simulink model "Control_test"  (R2014b)
settings: Solver=FixedStepDiscrete  StartTime=0.0  StopTime=Inf  FixedStep=0.001  RelTol=1e-3
PostLoadFcn:
  | , if any(exist('dsrtsu_mdlpostloadfcn', 'file') == [2, 3, 6]), try dsrtsu_mdlpostloadfcn('Execute', bdroot); catch fprintf('Error in PostLoadFcn (dsrtsu_mdlpostloadfcn) for model "%s":\n %s\n', bdroot, lasterr); end, end,
undefined symbols (not defined in the file or in its folder): dtLocal, slcm
libraries: rtican x163, simulink x14
(part 31 of 34)

== system Control_test/InputProcessing/VehicleCanProcessing/EMS2 ==
  Bus Creator : BusCreator  Inputs=19
  L_EMS2 : rtican/RTICAN Receive (RX)   Reserved1=[]  Reserved2=[]  Reserved3=[]  Reserved4=[]  SfcnMessage=[]  Msg_Struct=[]  BoardTypeNo=[]  BoardNo=[]  ChannelNo=[]  Parameters=[]  DialogFcn=[]  UnitName=[]  Revision=[]  UnitValues=[]  DSProperties=struct('RTI',struct('Version',uint32(5),'BlockType',struct('isSLSource',uint8(1),'isSLSink',uint8(1),'isHWSource',uint8(0),'isHWSink',uint8(0),'isSetup',uint8(0),'isInline',uint8(1),'isNonInline',uint8(0),'isInterrupt',uint8(0),'isChannelwise',uint8(0)),'IOBoardType','RTICAN','UnitType','MESSAGE','Identifier','RX','DialogType','MSVC','BlockSet','RTICAN','SlaveProcessor','CAN'))  RTIBlockInterface=struct('OutputPortsWidth',int32([1 1 1 1 1 1 1 1 1 1 1 1 1 1 1 1 1 1 1]),'OutputPortsActive',[1 1 1 1 1 1 1 1 1 1 1 1 1 1 1 1 1 1 1],'OutputPortsName',{{'PV_AV_CAN','TEMP_ENG','MAF_FAC_ALTI_MMV','VB_OFF_ACT','GP_CTL','CLU_ACK','OD_OFF_REQ','BRAKE_ACT','ACK_ES','ENG_CHR','CONF_MIL_FMY','ACC_ACT','TPS','ENG_VOL','MUL_CODE','CAN_VERS','CONF_TCU','OBD_FRF_ACK','TQ_STND'}},'OutputPortsDataType',{{'SS_DOUBLE','SS_DOUBLE','SS_DOUBLE','SS_DOUBLE','SS_DOUBLE','SS_DOUBLE','SS_DOUBLE','SS_DOUBLE','SS_DOUBLE','SS_DOUBLE','SS_DOUBLE','SS_DOUBLE','SS_DOUBLE','SS_DOUBLE','SS_DOUBLE','SS_DOUBLE','SS_DOUBLE','SS_DOUBLE','SS_DOUBLE'}},'OutputPortsLabel',{{'PV_AV_CAN','TEMP_ENG','MAF_FAC_ALTI_MMV','VB_OFF_ACT','GP_CTL','CLU_ACK','OD_OFF_REQ','BRAKE_ACT','ACK_ES','ENG_CHR','CONF_MIL_FMY','ACC_ACT','TPS','ENG_VOL','MUL_CODE','CAN_VERS','CONF_TCU','OBD_FRF_ACK','TQ_STND'}},'OutputPortsLabelMode','ON','InputPortsWidth',int32(0),'InputPortsActive',0,'DialogFcn','rtican_message_interface_gui','BlockDisplay',{{'','center'}},'IconTransparency','on','ParameterTunableNames',{{}},'InitLevel',3,'BlockName',struct('Token',{{'L_EMS2'}}),'SampleTime',{{-1}},'TriggerPort',{{'none'}},'EnablePort',{{'none'}})  RTIBlockParameters=struct('BoardTypeNo',{{1,'OFF',[]}},'BoardNo',{{1,'ON',[1 16]}},'ChannelNo',{{1,'ON',[1 2]}},'Parameters',{{struct('DataFileSupport',struct('DataFileSelectedMaster',1,'DataFileSelectedLocal',1,'DataFileName','c:\users\mpc_car\documents\github\mpc-car\controller\dbcfiles\hmc_can_for_ucb_v1.dbc|','DataFileDate',['21-Nov-2014 13:30:51'],'SelectedFile','c:\users\mpc_car\documents\github\mpc-car\dbcfiles\hmc_can_for_ucb_v2.dbc','InterfaceFcn','rtican_dbc_file_parser'),'Options',struct('StatusSelected',0,'TimeSelected',0,'DeltaTimeSelected',0,'BytePortSelected',0,'MessageLengthSelected',0,'TriggerPort',struct('Selected',0,'TriggerType',0),'UserCoding',struct('Selected',0,'InterfaceFile','UserDecodingFile','FcnName','UserDecodeFcn','InportSelected',0,'InportWidth',1,'OutportSelected',0,'OutportWidth',1),'EnablePortSelected',0,'SignalOnPortnameSelected',1,'UseRXService',0),'Message',struct('MsgOnBlocknameSelected',1,'MsgName','L_EMS2','MsgIdFormat',0,'MsgId',515,'MsgLength',8,'NumSignals',19,'SampleTime',-1,'Signal',struct('SgnName',{'PV_AV_CAN','TEMP_ENG','MAF_FAC_ALTI_MMV','VB_OFF_ACT','GP_CTL','CLU_ACK','OD_OFF_REQ','BRAKE_ACT','ACK_ES','ENG_CHR','CONF_MIL_FMY','ACC_ACT','TPS','ENG_VOL','MUL_CODE','CAN_VERS','CONF_TCU','OBD_FRF_ACK','TQ_STND'},'SgnStartBit',{0,8,16,24,25,27,28,29,31,32,36,39,40,48,56,58,58,58,58},'SgnLength',{8,8,8,1,2,1,1,2,1,4,3,1,8,8,2,6,6,6,6},'ByteLayout',{0,0,0,0,0,0,0,0,0,0,0,0,0,0,0,0,0,0,0},'Factor',{0.3906,0.75,0.00781,1,1,1,1,1,1,1,1,1,0.4694836,0.1,1,1,1,1,10},'Offset',{0,-48,0,0,0,0,0,0,0,0,0,0,-15.0234742,0,0,0,0,0,0},'SgnComment',{['In case of Delphi ECU, Output period tolerance(+1ms) will be applied to Engine Lamda3.'],['In case of Delphi ECU, Output period tolerance(+1ms) will be applied to Engine Lamda3.'],['In case of Delphi ECU, Output period tolerance(+1ms) will be applied to Engine Lamda3.'],['1. This signal is only for the gasoline system.' char(10) '2. In case of Delphi ECU, Output period tolerance(+1ms) will be applied to Engine Lamda3.'],['1. This signal is for the diesel engine system only.' char(10) '2. In case of Delphi ECU, Output period tolerance(+1ms) will be applied to Engine Lamda3.'],['1. This signal is for the diesel engine and ISG system installed vehicles only.' char(10) '2. In case of Delphi ECU, Output period tolerance(+1ms) will be applied to Engine Lamda3.'],['1. This signal is available in the auto cruise control system equiped vehicles only.' char(10) '2. In case of Delphi ECU, Output period tolerance(+1ms) will be applied to Engine Lamda3.'],['In case of Delphi ECU, Output period tolerance(+1ms) will be applied to Engine Lamda3.'],['In case of Delphi ECU, Output period tolerance(+1ms) will be applied to Engine Lamda3.'],['1. For the automatic variant coding at E.O.L : This signal value is valid 1.5sec later from initial IG-ON' char(10) '2. In case of Delphi ECU, Output period tolerance(+1ms) will be applied to Engine Lamda3.'],['1. This value represents a calibrated constant from the ECU.' char(10) '2. In case of Delphi ECU, Output period tolerance(+1ms) will be applied to Engine Lamda3.'],['1. There is signal relationship between ¡®ACC_ACT¡¯ and ¡®PV_AV_CAN¡¯. See ¡®PV_AV_CAN¡¯ signal description page.' char(10) '2. In case of Delphi ECU, Output period tolerance(+1ms) will be applied to Engine Lamda3.'],['1. In diesel engine system, there is a signal relationship between TPS and PV_AV_CAN. For the details, please see PV_AV_CAN signal description page. ' char(10) '2. In case of Delphi ECU, Output period tolerance(+1ms) will be applied to Engine Lamda3.'],['In case of Delphi ECU, Output period tolerance(+1ms) will be applied to Engine Lamda3.'],['In case of Delphi ECU, Output period tolerance(+1ms) will be applied to Engine Lamda3.'],['In case of Delphi ECU, Output period tolerance(+1ms) will be applied to Engine Lamda3.'],['1. For the automatic variant coding at E.O.L : This signal value is valid 1.5sec later from initial IG-ON' char(10) '2. In case of Delphi ECU, Output period tolerance(+1ms) will be applied to Engine Lamda3.'],['In case of Delphi ECU, Output period tolerance(+1ms) will be applied to Engine Lamda3.'],['1. In case of an engine which maximum engine torque is higher than 520Nm, this factor value is 15.' char(10) '2. In case of Delphi ECU, Output period tolerance(+1ms) will be applied to Engine Lamda3.']},'SgnUnit',{'%','¡É','','','','','','','','','','','%','liter','','','','','Nm'},'Min',{0,-48,0,0,0,0,0,0,0,0,0,0,-15.0234742,0,0,0,0,0,0},'Max',{99.603,143.25,1.99155,1,3,1,1,3,1,15,7,1,104.6948357,25.5,3,7.7,63,63,630},'SgnType',{0,0,0,0,0,0,0,0,0,0,0,0,0,0,1,2,2,2,2},'SLDataType',{'SS_DOUBLE','SS_DOUBLE','SS_DOUBLE','SS_DOUBLE','SS_DOUBLE','SS_DOUBLE','SS_DOUBLE','SS_DOUBLE','SS_DOUBLE','SS_DOUBLE','SS_DOUBLE','SS_DOUBLE','SS_DOUBLE','SS_DOUBLE','SS_DOUBLE','SS_DOUBLE','SS_DOUBLE','SS_DOUBLE','SS_DOUBLE'},'DataType',{0,0,0,0,0,0,0,0,0,0,0,0,0,0,0,0,0,0,0},'ModeValue',{-1,-1,-1,-1,-1,-1,-1,-1,-1,-1,-1,-1,-1,-1,-1,0,1,2,3}),'MsgIdNumFormat',0,'MsgComment',{{''}}),'Version',1.2,'general',struct('isFromLib',0)),'OFF',[]}},'GroupId',{{struct('Group',{{'RTICAN'}},'No',1,'Behavior',{{'NAMECHANGE'}},'BlockType',{{'SINK'}},'NameChangeFlag',0),'OFF',[]}},'SFcnRTICANMessage',{{struct('MsgType','RX','SFcnPortType','Scalar','MsgName','L_EMS2','MsgIdFormat','STD','MsgId',515,'MsgLength',8,'NumSignals',19,'SampleTime',-1,'Signal',struct('SgnName',{'PV_AV_CAN','TEMP_ENG','MAF_FAC_ALTI_MMV','VB_OFF_ACT','GP_CTL','CLU_ACK','OD_OFF_REQ','BRAKE_ACT','ACK_ES','ENG_CHR','CONF_MIL_FMY','ACC_ACT','TPS','ENG_VOL','MUL_CODE','CAN_VERS','CONF_TCU','OBD_FRF_ACK','TQ_STND'},'SgnStartBit',{0,8,16,24,25,27,28,29,31,32,36,39,40,48,56,58,58,58,58},'SgnLength',{8,8,8,1,2,1,1,2,1,4,3,1,8,8,2,6,6,6,6},'ByteLayout',{['little endian'],['little endian'],['little endian'],['little endian'],['little endian'],['little endian'],['little endian'],['little endian'],['little endian'],['little endian'],['little endian'],['little endian'],['little endian'],['little endian'],['little endian'],['little endian'],['little endian'],['little endian'],['little endian']},'Factor',{0.3906,0.75,0.00781,1,1,1,1,1,1,1,1,1,0.4694836,0.1,1,1,1,1,10},'Offset',{0,-48,0,0,0,0,0,0,0,0,0,0,-15.0234742,0,0,0,0,0,0},'SgnType',{'standard','standard','standard','standard','standard','standard','standard','standard','standard','standard','standard','standard','standard','standard','mode','mode-dependent','mode-dependent','mode-dependent','mode-dependent'},'SLDataType',{'SS_DOUBLE','SS_DOUBLE','SS_DOUBLE','SS_DOUBLE','SS_DOUBLE','SS_DOUBLE','SS_DOUBLE','SS_DOUBLE','SS_DOUBLE','SS_DOUBLE','SS_DOUBLE','SS_DOUBLE','SS_DOUBLE','SS_DOUBLE','SS_DOUBLE','SS_DOUBLE','SS_DOUBLE','SS_DOUBLE','SS_DOUBLE'},'DataType',{['unsigned int'],['unsigned int'],['unsigned int'],['unsigned int'],['unsigned int'],['unsigned int'],['unsigned int'],['unsigned int'],['unsigned int'],['unsigned int'],['unsigned int'],['unsigned int'],['unsigned int'],['unsigned int'],['unsigned int'],['unsigned int'],['unsigned int'],['unsigned int'],['unsigned int']},'ModeValue',{-1,-1,-1,-1,-1,-1,-1,-1,-1,-1,-1,-1,-1,-1,-1,0,1,2,3}),'StatusSelected','no','TimeSelected','no','DeltaTimeSelected','no','BytePortSelected','no','MessageLengthSelected','no','TriggerPort',struct('Selected','no','TriggerType',0),'UserCoding',struct('Selected','no','InterfaceFile','UserDecodingFile','FcnName','UserDecodeFcn','InportSelected','no','InportWidth',1,'OutportSelected','no','OutportWidth',1),'EnablePortSelected','no','UseRXService','no','BoardType','DS1','BoardNo',1,'ControllerNo',1),'OFF',[]}},'TLCFileName',{{'rtican_rx_message','OFF',[]}})  RTISFcnParameters=struct('SFcnRTICANMessage','struct','TLCFileName','char')  RTIBlockParaDefault=struct('BoardTypeNo',4302,'BoardNo',1,'ChannelNo',1,'Parameters',struct('DataFileSupport',struct('DataFileSelectedMaster',0,'DataFileSelectedLocal',0,'DataFileName','','DataFileDate','','SelectedFile',['<no file selected>']),'Options',struct('StatusSelected',1,'TimeSelected',1,'DeltaTimeSelected',1,'BytePortSelected',0,'MessageLengthSelected',0,'TriggerPort',struct('Selected',0,'TriggerType','rising'),'UserCoding',struct('Selected',0,'InterfaceFile','UserDecodingFile','FcnName','UserDecodeFcn','InportSelected',0,'InportWidth',1,'OutportSelected',0,'OutportWidth',1),'EnablePortSelected',0,'SignalOnPortnameSelected',1,'UseRXService',0),'Message',struct('MsgOnBlocknameSelected',0,'MsgName',['RX Message'],'MsgIdFormat',0,'MsgId',100,'MsgLength',8,'NumSignals',1,'SampleTime',-1,'Signal',struct('SgnName',['RX signal'],'SgnStartBit',0,'SgnLength',8,'SgnType',0,'ModeValue',-1,'DataType',0,'SLDataType','SS_DOUBLE','ByteLayout',0,'Factor',1,'Offset',0,'Min',0,'Max',255,'SgnComment',{{}},'SgnUnit',''),'MsgIdNumFormat',0,'MsgComment',{{''}}),'Version',1.2,'general',struct('isFromLib',1)),'GroupId',struct('Group',{{'RTICAN'}},'No',1,'Behavior',{{'NAMECHANGE'}},'BlockType',{{'SINK'}},'NameChangeFlag',0),'SFcnRTICANMessage',struct('MsgType','RX','MsgName',['RX Message'],'MsgIdFormat','STD','MsgId',100,'MsgLength',8,'NumSignals',1,'SampleTime',-1,'Signal',struct('SgnName',['RX signal'],'SgnStartBit',0,'SgnLength',8,'SgnType','standard','ModeValue',-1,'DataType',['unsigned int'],'ByteLayout',['little endian'],'SLDataType','SS_DOUBLE','Factor',1,'Offset',0),'StatusSelected','yes','TimeSelected','yes','DeltaTimeSelected','yes','BytePortSelected','no','MessageLengthSelected','no','EnablePortSelected','no','UserCoding',struct('Selected','no','InterfaceFile','UserDecodingFile','FcnName','UserDecodeFcn','InportSelected','no','InportWidth',1,'OutportSelected','no','OutportWidth',1),'TriggerPort',struct('Selected','no','TriggerType','rising'),'UseRXService','no','BoardType','DS4302','BoardNo',1,'ControllerNo',1,'SFcnPortType','Scalar'),'TLCFileName','rtican_rx_message')
      settings: AttributesFormatString=Group Id: RTICAN1\n
  EMS2_CAN : Outport
  wires:
  Bus Creator/1 -> EMS2_CAN/1  "EMS2_CAN"
  L_EMS2/1 -> Bus Creator/1  "PV_AV_CAN"
  L_EMS2/2 -> Bus Creator/2  "TEMP_ENG"
  L_EMS2/3 -> Bus Creator/3  "MAF_FAC_ALTI_MMV"
  L_EMS2/4 -> Bus Creator/4  "VB_OFF_ACT"
  L_EMS2/5 -> Bus Creator/5  "GP_CTL"
  L_EMS2/6 -> Bus Creator/6  "CLU_ACK"
  L_EMS2/7 -> Bus Creator/7  "OD_OFF_REQ"
  L_EMS2/8 -> Bus Creator/8  "BRAKE_ACT"
  L_EMS2/9 -> Bus Creator/9  "ACK_ES"
  L_EMS2/10 -> Bus Creator/10  "ENG_CHR"
  L_EMS2/11 -> Bus Creator/11  "CONF_MIL_FMY"
  L_EMS2/12 -> Bus Creator/12  "ACC_ACT"
  L_EMS2/13 -> Bus Creator/13  "TPS"
  L_EMS2/14 -> Bus Creator/14  "ENG_VOL"
  L_EMS2/15 -> Bus Creator/15  "MUL_CODE"
  L_EMS2/16 -> Bus Creator/16  "CAN_VERS"
  L_EMS2/17 -> Bus Creator/17  "CONF_TCU"
  L_EMS2/18 -> Bus Creator/18  "OBD_FRF_ACK"
  L_EMS2/19 -> Bus Creator/19  "TQ_STND"

== system Control_test/InputProcessing/VehicleCanProcessing/ESP2 ==
  Bus Creator : BusCreator  Inputs=12
  L_ESP2 : rtican/RTICAN Receive (RX)   Reserved1=[]  Reserved2=[]  Reserved3=[]  Reserved4=[]  SfcnMessage=[]  Msg_Struct=[]  BoardTypeNo=[]  BoardNo=[]  ChannelNo=[]  Parameters=[]  DialogFcn=[]  UnitName=[]  Revision=[]  UnitValues=[]  DSProperties=struct('RTI',struct('Version',uint32(5),'BlockType',struct('isSLSource',uint8(1),'isSLSink',uint8(1),'isHWSource',uint8(0),'isHWSink',uint8(0),'isSetup',uint8(0),'isInline',uint8(1),'isNonInline',uint8(0),'isInterrupt',uint8(0),'isChannelwise',uint8(0)),'IOBoardType','RTICAN','UnitType','MESSAGE','Identifier','RX','DialogType','MSVC','BlockSet','RTICAN','SlaveProcessor','CAN'))  RTIBlockInterface=struct('OutputPortsWidth',int32([1 1 1 1 1 1 1 1 1 1 1 1]),'OutputPortsActive',[1 1 1 1 1 1 1 1 1 1 1 1],'OutputPortsName',{{'LAT_ACCEL','LONG_ACCEL_STAT','LAT_ACCEL_STAT','LONG_ACCEL_DIAG','CYL_PRES_STAT','CYL_PRESS_DIAG','YAW_RATE','YAW_RATE_STAT','LAT_ACCEL_DIAG','YAW_RATE_DIAG','LONG_ACCEL','CYL_PRES'}},'OutputPortsDataType',{{'SS_DOUBLE','SS_DOUBLE','SS_DOUBLE','SS_DOUBLE','SS_DOUBLE','SS_DOUBLE','SS_DOUBLE','SS_DOUBLE','SS_DOUBLE','SS_DOUBLE','SS_DOUBLE','SS_DOUBLE'}},'OutputPortsLabel',{{'LAT_ACCEL','LONG_ACCEL_STAT','LAT_ACCEL_STAT','LONG_ACCEL_DIAG','CYL_PRES_STAT','CYL_PRESS_DIAG','YAW_RATE','YAW_RATE_STAT','LAT_ACCEL_DIAG','YAW_RATE_DIAG','LONG_ACCEL','CYL_PRES'}},'OutputPortsLabelMode','ON','InputPortsWidth',int32(0),'InputPortsActive',0,'DialogFcn','rtican_message_interface_gui','BlockDisplay',{{'','center'}},'IconTransparency','on','ParameterTunableNames',{{}},'InitLevel',3,'BlockName',struct('Token',{{'L_ESP2'}}),'SampleTime',{{-1}},'TriggerPort',{{'none'}},'EnablePort',{{'none'}})  RTIBlockParameters=struct('BoardTypeNo',{{1,'OFF',[]}},'BoardNo',{{1,'ON',[1 16]}},'ChannelNo',{{1,'ON',[1 2]}},'Parameters',{{struct('DataFileSupport',struct('DataFileSelectedMaster',1,'DataFileSelectedLocal',1,'DataFileName','c:\users\mpc_car\documents\github\mpc-car\controller\dbcfiles\hmc_can_for_ucb_v1.dbc|','DataFileDate',['21-Nov-2014 13:30:51'],'SelectedFile','c:\users\mpc_car\documents\github\mpc-car\dbcfiles\hmc_can_for_ucb_v2.dbc','InterfaceFcn','rtican_dbc_file_parser'),'Options',struct('StatusSelected',0,'TimeSelected',0,'DeltaTimeSelected',0,'BytePortSelected',0,'MessageLengthSelected',0,'TriggerPort',struct('Selected',0,'TriggerType',0),'UserCoding',struct('Selected',0,'InterfaceFile','UserDecodingFile','FcnName','UserDecodeFcn','InportSelected',0,'InportWidth',1,'OutportSelected',0,'OutportWidth',1),'EnablePortSelected',0,'SignalOnPortnameSelected',1,'UseRXService',0),'Message',struct('MsgOnBlocknameSelected',1,'MsgName','L_ESP2','MsgIdFormat',0,'MsgId',516,'MsgLength',8,'NumSignals',12,'SampleTime',-1,'Signal',struct('SgnName',{'LAT_ACCEL','LONG_ACCEL_STAT','LAT_ACCEL_STAT','LONG_ACCEL_DIAG','CYL_PRES_STAT','CYL_PRESS_DIAG','YAW_RATE','YAW_RATE_STAT','LAT_ACCEL_DIAG','YAW_RATE_DIAG','LONG_ACCEL','CYL_PRES'},'SgnStartBit',{0,11,12,13,14,15,16,29,30,31,32,48},'SgnLength',{11,1,1,1,1,1,13,1,1,1,11,12},'ByteLayout',{0,0,0,0,0,0,0,0,0,0,0,0},'Factor',{0.01,1,1,1,1,1,0.01,1,1,1,0.01,0.1},'Offset',{-10.23,0,0,0,0,0,-40.95,0,0,0,-10.23,0},'SgnComment',{'','','','','','','','','','','',''},'SgnUnit',{'m/s^2','','','','','','¢ª/s','','','','m/s^2','bar'},'Min',{-10.23,0,0,0,0,0,-40.95,0,0,0,-10.23,0},'Max',{10.24,1,1,1,1,1,40.96,1,1,1,10.24,409.5},'SgnType',{0,0,0,0,0,0,0,0,0,0,0,0},'SLDataType',{'SS_DOUBLE','SS_DOUBLE','SS_DOUBLE','SS_DOUBLE','SS_DOUBLE','SS_DOUBLE','SS_DOUBLE','SS_DOUBLE','SS_DOUBLE','SS_DOUBLE','SS_DOUBLE','SS_DOUBLE'},'DataType',{0,0,0,0,0,0,0,0,0,0,0,0},'ModeValue',{-1,-1,-1,-1,-1,-1,-1,-1,-1,-1,-1,-1}),'MsgIdNumFormat',0,'MsgComment',{{''}}),'Version',1.2,'general',struct('isFromLib',0)),'OFF',[]}},'GroupId',{{struct('Group',{{'RTICAN'}},'No',1,'Behavior',{{'NAMECHANGE'}},'BlockType',{{'SINK'}},'NameChangeFlag',0),'OFF',[]}},'SFcnRTICANMessage',{{struct('MsgType','RX','SFcnPortType','Scalar','MsgName','L_ESP2','MsgIdFormat','STD','MsgId',516,'MsgLength',8,'NumSignals',12,'SampleTime',-1,'Signal',struct('SgnName',{'LAT_ACCEL','LONG_ACCEL_STAT','LAT_ACCEL_STAT','LONG_ACCEL_DIAG','CYL_PRES_STAT','CYL_PRESS_DIAG','YAW_RATE','YAW_RATE_STAT','LAT_ACCEL_DIAG','YAW_RATE_DIAG','LONG_ACCEL','CYL_PRES'},'SgnStartBit',{0,11,12,13,14,15,16,29,30,31,32,48},'SgnLength',{11,1,1,1,1,1,13,1,1,1,11,12},'ByteLayout',{['little endian'],['little endian'],['little endian'],['little endian'],['little endian'],['little endian'],['little endian'],['little endian'],['little endian'],['little endian'],['little endian'],['little endian']},'Factor',{0.01,1,1,1,1,1,0.01,1,1,1,0.01,0.1},'Offset',{-10.23,0,0,0,0,0,-40.95,0,0,0,-10.23,0},'SgnType',{'standard','standard','standard','standard','standard','standard','standard','standard','standard','standard','standard','standard'},'SLDataType',{'SS_DOUBLE','SS_DOUBLE','SS_DOUBLE','SS_DOUBLE','SS_DOUBLE','SS_DOUBLE','SS_DOUBLE','SS_DOUBLE','SS_DOUBLE','SS_DOUBLE','SS_DOUBLE','SS_DOUBLE'},'DataType',{['unsigned int'],['unsigned int'],['unsigned int'],['unsigned int'],['unsigned int'],['unsigned int'],['unsigned int'],['unsigned int'],['unsigned int'],['unsigned int'],['unsigned int'],['unsigned int']},'ModeValue',{-1,-1,-1,-1,-1,-1,-1,-1,-1,-1,-1,-1}),'StatusSelected','no','TimeSelected','no','DeltaTimeSelected','no','BytePortSelected','no','MessageLengthSelected','no','TriggerPort',struct('Selected','no','TriggerType',0),'UserCoding',struct('Selected','no','InterfaceFile','UserDecodingFile','FcnName','UserDecodeFcn','InportSelected','no','InportWidth',1,'OutportSelected','no','OutportWidth',1),'EnablePortSelected','no','UseRXService','no','BoardType','DS1','BoardNo',1,'ControllerNo',1),'OFF',[]}},'TLCFileName',{{'rtican_rx_message','OFF',[]}})  RTISFcnParameters=struct('SFcnRTICANMessage','struct','TLCFileName','char')  RTIBlockParaDefault=struct('BoardTypeNo',4302,'BoardNo',1,'ChannelNo',1,'Parameters',struct('DataFileSupport',struct('DataFileSelectedMaster',0,'DataFileSelectedLocal',0,'DataFileName','','DataFileDate','','SelectedFile',['<no file selected>']),'Options',struct('StatusSelected',1,'TimeSelected',1,'DeltaTimeSelected',1,'BytePortSelected',0,'MessageLengthSelected',0,'TriggerPort',struct('Selected',0,'TriggerType','rising'),'UserCoding',struct('Selected',0,'InterfaceFile','UserDecodingFile','FcnName','UserDecodeFcn','InportSelected',0,'InportWidth',1,'OutportSelected',0,'OutportWidth',1),'EnablePortSelected',0,'SignalOnPortnameSelected',1,'UseRXService',0),'Message',struct('MsgOnBlocknameSelected',0,'MsgName',['RX Message'],'MsgIdFormat',0,'MsgId',100,'MsgLength',8,'NumSignals',1,'SampleTime',-1,'Signal',struct('SgnName',['RX signal'],'SgnStartBit',0,'SgnLength',8,'SgnType',0,'ModeValue',-1,'DataType',0,'SLDataType','SS_DOUBLE','ByteLayout',0,'Factor',1,'Offset',0,'Min',0,'Max',255,'SgnComment',{{}},'SgnUnit',''),'MsgIdNumFormat',0,'MsgComment',{{''}}),'Version',1.2,'general',struct('isFromLib',1)),'GroupId',struct('Group',{{'RTICAN'}},'No',1,'Behavior',{{'NAMECHANGE'}},'BlockType',{{'SINK'}},'NameChangeFlag',0),'SFcnRTICANMessage',struct('MsgType','RX','MsgName',['RX Message'],'MsgIdFormat','STD','MsgId',100,'MsgLength',8,'NumSignals',1,'SampleTime',-1,'Signal',struct('SgnName',['RX signal'],'SgnStartBit',0,'SgnLength',8,'SgnType','standard','ModeValue',-1,'DataType',['unsigned int'],'ByteLayout',['little endian'],'SLDataType','SS_DOUBLE','Factor',1,'Offset',0),'StatusSelected','yes','TimeSelected','yes','DeltaTimeSelected','yes','BytePortSelected','no','MessageLengthSelected','no','EnablePortSelected','no','UserCoding',struct('Selected','no','InterfaceFile','UserDecodingFile','FcnName','UserDecodeFcn','InportSelected','no','InportWidth',1,'OutportSelected','no','OutportWidth',1),'TriggerPort',struct('Selected','no','TriggerType','rising'),'UseRXService','no','BoardType','DS4302','BoardNo',1,'ControllerNo',1,'SFcnPortType','Scalar'),'TLCFileName','rtican_rx_message')
      settings: AttributesFormatString=Group Id: RTICAN1\n
  ESP2_CAN : Outport
  wires:
  Bus Creator/1 -> ESP2_CAN/1  "ESP2_CAN"
  L_ESP2/1 -> Bus Creator/1  "LAT_ACCEL"
  L_ESP2/2 -> Bus Creator/2  "LONG_ACCEL_STAT"
  L_ESP2/3 -> Bus Creator/3  "LAT_ACCEL_STAT"
  L_ESP2/4 -> Bus Creator/4  "LONG_ACCEL_DIAG"
  L_ESP2/5 -> Bus Creator/5  "CYL_PRES_STAT"
  L_ESP2/6 -> Bus Creator/6  "CYL_PRESS_DIAG"
  L_ESP2/7 -> Bus Creator/7  "YAW_RATE"
  L_ESP2/8 -> Bus Creator/8  "YAW_RATE_STAT"
  L_ESP2/9 -> Bus Creator/9  "LAT_ACCEL_DIAG"
  L_ESP2/10 -> Bus Creator/10  "YAW_RATE_DIAG"
  L_ESP2/11 -> Bus Creator/11  "LONG_ACCEL"
  L_ESP2/12 -> Bus Creator/12  "CYL_PRES"

== system Control_test/InputProcessing/VehicleCanProcessing/ESP2Processing ==
  In1 : Inport
  Bus Creator3 : BusCreator  Inputs=12
  Bus Selector3 : BusSelector  OutputSignals=LAT_ACCEL,LAT_ACCEL_STAT,LAT_ACCEL_DIAG,LONG_ACCEL,LONG_ACCEL_STAT,LONG_ACCEL_DIAG,CYL_PRES,CYL_PRES_STAT,CYL_PRESS_DIAG,YAW_RATE,YAW_RATE_STAT,YAW_RATE_DIAG
  ESP2 Processing : Subsystem
  Out1 : Outport
  tag scope: ipLongAccel=global
  wires:
  Bus Selector3/1 -> ESP2 Processing/1(LAT_ACCEL_CAN)  "<LAT_ACCEL>"
  Bus Selector3/2 -> ESP2 Processing/2(LAT_ACCEL_STAT_CAN)  "<LAT_ACCEL_STAT>"
  Bus Selector3/3 -> ESP2 Processing/3(LAT_ACCEL_DIAG_CAN)  "<LAT_ACCEL_DIAG>"
  Bus Selector3/4 -> ESP2 Processing/4(LONG_ACCEL_CAN)  "<LONG_ACCEL>"
  Bus Selector3/5 -> ESP2 Processing/5(LONG_ACCEL_STAT_CAN)  "<LONG_ACCEL_STAT>"
  Bus Selector3/6 -> ESP2 Processing/6(LONG_ACCEL_DIAG_CAN)  "<LONG_ACCEL_DIAG>"
  Bus Selector3/7 -> ESP2 Processing/7(CYL_PRES_CAN)  "<CYL_PRES>"
  Bus Selector3/8 -> ESP2 Processing/8(CYL_PRES_STAT_CAN)  "<CYL_PRES_STAT>"
  Bus Selector3/9 -> ESP2 Processing/9(CYL_PRES_DIAG_CAN)  "<CYL_PRESS_DIAG>"
  Bus Selector3/10 -> ESP2 Processing/10(YAW_RATE_CAN)  "<YAW_RATE>"
  Bus Selector3/11 -> ESP2 Processing/11(YAW_RATE_STAT_CAN)  "<YAW_RATE_STAT>"
  Bus Selector3/12 -> ESP2 Processing/12(YAW_RATE_DIAG_CAN)  "<YAW_RATE_DIAG>"
  ESP2 Processing/1(ipLatAccel [m/s2]) -> Bus Creator3/1
  ESP2 Processing/2(ipLatAccelFail) -> Bus Creator3/2
  ESP2 Processing/3(ipLatAccelDiag) -> Bus Creator3/3
  ESP2 Processing/4(ipLongAccel [m/s2]) -> [ipLongAccel], Bus Creator3/4
  ESP2 Processing/5(ipLongAccelFail) -> Bus Creator3/5
  ESP2 Processing/6(ipLongAccelDiag) -> Bus Creator3/6
  ESP2 Processing/7(ipMsCylPress [bar]) -> Bus Creator3/7
  ESP2 Processing/8(ipMsCylPressFail) -> Bus Creator3/8
  ESP2 Processing/9(ipMsCylPressDiag) -> Bus Creator3/9
  ESP2 Processing/10(ipYawRate [deg/s]) -> Bus Creator3/10
  ESP2 Processing/11(ipYawRateFail) -> Bus Creator3/11
  ESP2 Processing/12(ipYawRateDiag) -> Bus Creator3/12
  Bus Creator3/1 -> Out1/1  "ESP2Data"
  In1/1 -> Bus Selector3/1

== system Control_test/InputProcessing/VehicleCanProcessing/MDPS2 ==
  Bus Creator : BusCreator  Inputs=5
  L_MDPS2 : rtican/RTICAN Receive (RX)   Reserved1=[]  Reserved2=[]  Reserved3=[]  Reserved4=[]  SfcnMessage=[]  Msg_Struct=[]  BoardTypeNo=[]  BoardNo=[]  ChannelNo=[]  Parameters=[]  DialogFcn=[]  UnitName=[]  Revision=[]  UnitValues=[]  DSProperties=struct('RTI',struct('Version',uint32(5),'BlockType',struct('isSLSource',uint8(1),'isSLSink',uint8(1),'isHWSource',uint8(0),'isHWSink',uint8(0),'isSetup',uint8(0),'isInline',uint8(1),'isNonInline',uint8(0),'isInterrupt',uint8(0),'isChannelwise',uint8(0)),'IOBoardType','RTICAN','UnitType','MESSAGE','Identifier','RX','DialogType','MSVC','BlockSet','RTICAN','SlaveProcessor','CAN'))  RTIBlockInterface=struct('OutputPortsWidth',int32([1 1 1 1 1]),'OutputPortsActive',[1 1 1 1 1],'OutputPortsName',{{'CR_Mdps_DrvTq','CR_Mdps_StrAng','CF_Mdps_AliveCnt','CF_Mdps_Stat','CF_Mdps_Chksum'}},'OutputPortsDataType',{{'SS_DOUBLE','SS_DOUBLE','SS_DOUBLE','SS_DOUBLE','SS_DOUBLE'}},'OutputPortsLabel',{{'CR_Mdps_DrvTq','CR_Mdps_StrAng','CF_Mdps_AliveCnt','CF_Mdps_Stat','CF_Mdps_Chksum'}},'OutputPortsLabelMode','ON','InputPortsWidth',int32(0),'InputPortsActive',0,'DialogFcn','rtican_message_interface_gui','BlockDisplay',{{'','center'}},'IconTransparency','on','ParameterTunableNames',{{}},'InitLevel',3,'BlockName',struct('Token',{{'L_MDPS2'}}),'SampleTime',{{-1}},'TriggerPort',{{'none'}},'EnablePort',{{'none'}})  RTIBlockParameters=struct('BoardTypeNo',{{1,'OFF',[]}},'BoardNo',{{1,'ON',[1 16]}},'ChannelNo',{{1,'ON',[1 2]}},'Parameters',{{struct('DataFileSupport',struct('DataFileSelectedMaster',1,'DataFileSelectedLocal',1,'DataFileName',['c:\users\mpc lab\documents\github\controller\dbcfiles\hmc_can_for_ucb_v2.dbc|'],'DataFileDate',{{{['10-Feb-2015 13:24:58']}}},'SelectedFile','..\..\..\dbcfiles\hmc_can_for_ucb_v2.dbc','InterfaceFcn','rtican_dbc_file_parser'),'Options',struct('StatusSelected',0,'TimeSelected',0,'DeltaTimeSelected',0,'BytePortSelected',0,'MessageLengthSelected',0,'TriggerPort',struct('Selected',0,'TriggerType',0),'UserCoding',struct('Selected',0,'InterfaceFile','UserDecodingFile','FcnName','UserDecodeFcn','InportSelected',0,'InportWidth',1,'OutportSelected',0,'OutportWidth',1),'EnablePortSelected',0,'SignalOnPortnameSelected',1,'UseRXService',0),'Message',struct('MsgOnBlocknameSelected',1,'MsgName','L_MDPS2','MsgIdFormat',0,'MsgId',517,'MsgLength',8,'NumSignals',5,'SampleTime',-1,'Signal',struct('SgnName',{'CR_Mdps_DrvTq','CR_Mdps_StrAng','CF_Mdps_AliveCnt','CF_Mdps_Stat','CF_Mdps_Chksum'},'SgnStartBit',{0,16,40,48,56},'SgnLength',{12,16,8,4,8},'SgnType',{0,0,0,0,0},'ModeValue',{-1,-1,-1,-1,-1},'DataType',{0,1,0,0,0},'ByteLayout',{0,0,0,0,0},'Factor',{0.01,0.1,1,1,1},'Offset',{-20.48,0,0,0,0},'SgnComment',{{''},{''},{''},{''},{''}},'SgnUnit',{'','Degree','','',''},'Min',{-20.48,-3276.8,0,0,0},'Max',{20.46,3276.7,255,15,255},'SLDataType',{'SS_DOUBLE','SS_DOUBLE','SS_DOUBLE','SS_DOUBLE','SS_DOUBLE'}),'MsgIdNumFormat',0,'MsgComment',{{''}}),'Version',1.2,'general',struct('isFromLib',0)),'OFF',[]}},'GroupId',{{struct('Group',{{'RTICAN'}},'No',1,'Behavior',{{'NAMECHANGE'}},'BlockType',{{'SINK'}},'NameChangeFlag',0),'OFF',[]}},'SFcnRTICANMessage',{{struct('MsgType','RX','SFcnPortType','Scalar','MsgName','L_MDPS2','MsgIdFormat','STD','MsgId',517,'MsgLength',8,'NumSignals',5,'SampleTime',-1,'Signal',struct('SgnName',{'CR_Mdps_DrvTq','CR_Mdps_StrAng','CF_Mdps_AliveCnt','CF_Mdps_Stat','CF_Mdps_Chksum'},'SgnStartBit',{0,16,40,48,56},'SgnLength',{12,16,8,4,8},'SgnType',{'standard','standard','standard','standard','standard'},'ModeValue',{-1,-1,-1,-1,-1},'DataType',{['unsigned int'],['signed int'],['unsigned int'],['unsigned int'],['unsigned int']},'ByteLayout',{['little endian'],['little endian'],['little endian'],['little endian'],['little endian']},'Factor',{0.01,0.1,1,1,1},'Offset',{-20.48,0,0,0,0},'SLDataType',{'SS_DOUBLE','SS_DOUBLE','SS_DOUBLE','SS_DOUBLE','SS_DOUBLE'}),'StatusSelected','no','TimeSelected','no','DeltaTimeSelected','no','BytePortSelected','no','MessageLengthSelected','no','TriggerPort',struct('Selected','no','TriggerType',0),'UserCoding',struct('Selected','no','InterfaceFile','UserDecodingFile','FcnName','UserDecodeFcn','InportSelected','no','InportWidth',1,'OutportSelected','no','OutportWidth',1),'EnablePortSelected','no','UseRXService','no','BoardType','DS1','BoardNo',1,'ControllerNo',1),'OFF',[]}},'TLCFileName',{{'rtican_rx_message','OFF',[]}})  RTISFcnParameters=struct('SFcnRTICANMessage','struct','TLCFileName','char')  RTIBlockParaDefault=struct('BoardTypeNo',4302,'BoardNo',1,'ChannelNo',1,'Parameters',struct('DataFileSupport',struct('DataFileSelectedMaster',0,'DataFileSelectedLocal',0,'DataFileName','','DataFileDate','','SelectedFile',['<no file selected>']),'Options',struct('StatusSelected',1,'TimeSelected',1,'DeltaTimeSelected',1,'BytePortSelected',0,'MessageLengthSelected',0,'TriggerPort',struct('Selected',0,'TriggerType','rising'),'UserCoding',struct('Selected',0,'InterfaceFile','UserDecodingFile','FcnName','UserDecodeFcn','InportSelected',0,'InportWidth',1,'OutportSelected',0,'OutportWidth',1),'EnablePortSelected',0,'SignalOnPortnameSelected',1,'UseRXService',0),'Message',struct('MsgOnBlocknameSelected',0,'MsgName',['RX Message'],'MsgIdFormat',0,'MsgId',100,'MsgLength',8,'NumSignals',1,'SampleTime',-1,'Signal',struct('SgnName',['RX signal'],'SgnStartBit',0,'SgnLength',8,'SgnType',0,'ModeValue',-1,'DataType',0,'SLDataType','SS_DOUBLE','ByteLayout',0,'Factor',1,'Offset',0,'Min',0,'Max',255,'SgnComment',{{}},'SgnUnit',''),'MsgIdNumFormat',0,'MsgComment',{{''}}),'Version',1.2,'general',struct('isFromLib',1)),'GroupId',struct('Group',{{'RTICAN'}},'No',1,'Behavior',{{'NAMECHANGE'}},'BlockType',{{'SINK'}},'NameChangeFlag',0),'SFcnRTICANMessage',struct('MsgType','RX','MsgName',['RX Message'],'MsgIdFormat','STD','MsgId',100,'MsgLength',8,'NumSignals',1,'SampleTime',-1,'Signal',struct('SgnName',['RX signal'],'SgnStartBit',0,'SgnLength',8,'SgnType','standard','ModeValue',-1,'DataType',['unsigned int'],'ByteLayout',['little endian'],'SLDataType','SS_DOUBLE','Factor',1,'Offset',0),'StatusSelected','yes','TimeSelected','yes','DeltaTimeSelected','yes','BytePortSelected','no','MessageLengthSelected','no','EnablePortSelected','no','UserCoding',struct('Selected','no','InterfaceFile','UserDecodingFile','FcnName','UserDecodeFcn','InportSelected','no','InportWidth',1,'OutportSelected','no','OutportWidth',1),'TriggerPort',struct('Selected','no','TriggerType','rising'),'UseRXService','no','BoardType','DS4302','BoardNo',1,'ControllerNo',1,'SFcnPortType','Scalar'),'TLCFileName','rtican_rx_message')
      settings: AttributesFormatString=Group Id: RTICAN1\n
  MDPS2_CAN : Outport
  wires:
  Bus Creator/1 -> MDPS2_CAN/1  "MDPS2"
  L_MDPS2/1 -> Bus Creator/1  "CR_Mdps_DrvTq"
  L_MDPS2/2 -> Bus Creator/2  "CR_Mdps_StrAng"
  L_MDPS2/3 -> Bus Creator/3  "CF_Mdps_AliveCnt"
  L_MDPS2/4 -> Bus Creator/4  "CF_Mdps_Stat"
  L_MDPS2/5 -> Bus Creator/5  "CF_Mdps_Chksum"

== system Control_test/InputProcessing/VehicleCanProcessing/MDPS2 Processing ==
  In1 : Inport
  Out1 : Outport
  wires:
  In1/1 -> Out1/1  "MDPS2Data"

== system Control_test/InputProcessing/VehicleCanProcessing/MDPS3 ==
  Bus Creator : BusCreator  Inputs=7
  L_MDPS3 : rtican/RTICAN Receive (RX)   Reserved1=[]  Reserved2=[]  Reserved3=[]  Reserved4=[]  SfcnMessage=[]  Msg_Struct=[]  BoardTypeNo=[]  BoardNo=[]  ChannelNo=[]  Parameters=[]  DialogFcn=[]  UnitName=[]  Revision=[]  UnitValues=[]  DSProperties=struct('RTI',struct('Version',uint32(5),'BlockType',struct('isSLSource',uint8(1),'isSLSink',uint8(1),'isHWSource',uint8(0),'isHWSink',uint8(0),'isSetup',uint8(0),'isInline',uint8(1),'isNonInline',uint8(0),'isInterrupt',uint8(0),'isChannelwise',uint8(0)),'IOBoardType','RTICAN','UnitType','MESSAGE','Identifier','RX','DialogType','MSVC','BlockSet','RTICAN','SlaveProcessor','CAN'))  RTIBlockInterface=struct('OutputPortsWidth',int32([1 1 1 1 1 1 1]),'OutputPortsActive',[1 1 1 1 1 1 1],'OutputPortsName',{{'CF_Mdps_MsgCount3','CR_Mdps_StrColTq','CF_Mdps_ToiFlt','CF_Mdps_ToiActive','CF_Mdps_FailStat','CF_Mdps_ToiUnavail','CF_Mdps_Chksum3'}},'OutputPortsDataType',{{'SS_DOUBLE','SS_DOUBLE','SS_DOUBLE','SS_DOUBLE','SS_DOUBLE','SS_DOUBLE','SS_DOUBLE'}},'OutputPortsLabel',{{'CF_Mdps_MsgCount3','CR_Mdps_StrColTq','CF_Mdps_ToiFlt','CF_Mdps_ToiActive','CF_Mdps_FailStat','CF_Mdps_ToiUnavail','CF_Mdps_Chksum3'}},'OutputPortsLabelMode','ON','InputPortsWidth',int32(0),'InputPortsActive',0,'DialogFcn','rtican_message_interface_gui','BlockDisplay',{{'','center'}},'IconTransparency','on','ParameterTunableNames',{{}},'InitLevel',3,'BlockName',struct('Token',{{'L_MDPS3'}}),'SampleTime',{{-1}},'TriggerPort',{{'none'}},'EnablePort',{{'none'}})  RTIBlockParameters=struct('BoardTypeNo',{{1,'OFF',[]}},'BoardNo',{{1,'ON',[1 16]}},'ChannelNo',{{1,'ON',[1 2]}},'Parameters',{{struct('DataFileSupport',struct('DataFileSelectedMaster',1,'DataFileSelectedLocal',1,'DataFileName','c:\users\mpc_car\documents\github\mpc-car\controller\dbcfiles\hmc_can_for_ucb_v1.dbc|','DataFileDate',['21-Nov-2014 13:30:51'],'SelectedFile','c:\users\mpc_car\documents\github\mpc-car\dbcfiles\hmc_can_for_ucb_v2.dbc','InterfaceFcn','rtican_dbc_file_parser'),'Options',struct('StatusSelected',0,'TimeSelected',0,'DeltaTimeSelected',0,'BytePortSelected',0,'MessageLengthSelected',0,'TriggerPort',struct('Selected',0,'TriggerType',0),'UserCoding',struct('Selected',0,'InterfaceFile','UserDecodingFile','FcnName','UserDecodeFcn','InportSelected',0,'InportWidth',1,'OutportSelected',0,'OutportWidth',1),'EnablePortSelected',0,'SignalOnPortnameSelected',1,'UseRXService',0),'Message',struct('MsgOnBlocknameSelected',1,'MsgName','L_MDPS3','MsgIdFormat',0,'MsgId',518,'MsgLength',8,'NumSignals',7,'SampleTime',-1,'Signal',struct('SgnName',{'CF_Mdps_MsgCount3','CR_Mdps_StrColTq','CF_Mdps_ToiFlt','CF_Mdps_ToiActive','CF_Mdps_FailStat','CF_Mdps_ToiUnavail','CF_Mdps_Chksum3'},'SgnStartBit',{0,8,19,20,21,22,24},'SgnLength',{8,11,1,1,1,1,8},'ByteLayout',{0,0,0,0,0,0,0},'Factor',{1,0.0078125,1,1,1,1,1},'Offset',{0,-8,0,0,0,0,0},'SgnComment',{'','','','','','',''},'SgnUnit',{'','Nm','','','','',''},'Min',{0,-8,0,0,0,0,0},'Max',{255,7.9921875,1,1,1,1,255},'SgnType',{0,0,0,0,0,0,0},'SLDataType',{'SS_DOUBLE','SS_DOUBLE','SS_DOUBLE','SS_DOUBLE','SS_DOUBLE','SS_DOUBLE','SS_DOUBLE'},'DataType',{0,0,0,0,0,0,0},'ModeValue',{-1,-1,-1,-1,-1,-1,-1}),'MsgIdNumFormat',0,'MsgComment',{{''}}),'Version',1.2,'general',struct('isFromLib',0)),'OFF',[]}},'GroupId',{{struct('Group',{{'RTICAN'}},'No',1,'Behavior',{{'NAMECHANGE'}},'BlockType',{{'SINK'}},'NameChangeFlag',0),'OFF',[]}},'SFcnRTICANMessage',{{struct('MsgType','RX','SFcnPortType','Scalar','MsgName','L_MDPS3','MsgIdFormat','STD','MsgId',518,'MsgLength',8,'NumSignals',7,'SampleTime',-1,'Signal',struct('SgnName',{'CF_Mdps_MsgCount3','CR_Mdps_StrColTq','CF_Mdps_ToiFlt','CF_Mdps_ToiActive','CF_Mdps_FailStat','CF_Mdps_ToiUnavail','CF_Mdps_Chksum3'},'SgnStartBit',{0,8,19,20,21,22,24},'SgnLength',{8,11,1,1,1,1,8},'ByteLayout',{['little endian'],['little endian'],['little endian'],['little endian'],['little endian'],['little endian'],['little endian']},'Factor',{1,0.0078125,1,1,1,1,1},'Offset',{0,-8,0,0,0,0,0},'SgnType',{'standard','standard','standard','standard','standard','standard','standard'},'SLDataType',{'SS_DOUBLE','SS_DOUBLE','SS_DOUBLE','SS_DOUBLE','SS_DOUBLE','SS_DOUBLE','SS_DOUBLE'},'DataType',{['unsigned int'],['unsigned int'],['unsigned int'],['unsigned int'],['unsigned int'],['unsigned int'],['unsigned int']},'ModeValue',{-1,-1,-1,-1,-1,-1,-1}),'StatusSelected','no','TimeSelected','no','DeltaTimeSelected','no','BytePortSelected','no','MessageLengthSelected','no','TriggerPort',struct('Selected','no','TriggerType',0),'UserCoding',struct('Selected','no','InterfaceFile','UserDecodingFile','FcnName','UserDecodeFcn','InportSelected','no','InportWidth',1,'OutportSelected','no','OutportWidth',1),'EnablePortSelected','no','UseRXService','no','BoardType','DS1','BoardNo',1,'ControllerNo',1),'OFF',[]}},'TLCFileName',{{'rtican_rx_message','OFF',[]}})  RTISFcnParameters=struct('SFcnRTICANMessage','struct','TLCFileName','char')  RTIBlockParaDefault=struct('BoardTypeNo',4302,'BoardNo',1,'ChannelNo',1,'Parameters',struct('DataFileSupport',struct('DataFileSelectedMaster',0,'DataFileSelectedLocal',0,'DataFileName','','DataFileDate','','SelectedFile',['<no file selected>']),'Options',struct('StatusSelected',1,'TimeSelected',1,'DeltaTimeSelected',1,'BytePortSelected',0,'MessageLengthSelected',0,'TriggerPort',struct('Selected',0,'TriggerType','rising'),'UserCoding',struct('Selected',0,'InterfaceFile','UserDecodingFile','FcnName','UserDecodeFcn','InportSelected',0,'InportWidth',1,'OutportSelected',0,'OutportWidth',1),'EnablePortSelected',0,'SignalOnPortnameSelected',1,'UseRXService',0),'Message',struct('MsgOnBlocknameSelected',0,'MsgName',['RX Message'],'MsgIdFormat',0,'MsgId',100,'MsgLength',8,'NumSignals',1,'SampleTime',-1,'Signal',struct('SgnName',['RX signal'],'SgnStartBit',0,'SgnLength',8,'SgnType',0,'ModeValue',-1,'DataType',0,'SLDataType','SS_DOUBLE','ByteLayout',0,'Factor',1,'Offset',0,'Min',0,'Max',255,'SgnComment',{{}},'SgnUnit',''),'MsgIdNumFormat',0,'MsgComment',{{''}}),'Version',1.2,'general',struct('isFromLib',1)),'GroupId',struct('Group',{{'RTICAN'}},'No',1,'Behavior',{{'NAMECHANGE'}},'BlockType',{{'SINK'}},'NameChangeFlag',0),'SFcnRTICANMessage',struct('MsgType','RX','MsgName',['RX Message'],'MsgIdFormat','STD','MsgId',100,'MsgLength',8,'NumSignals',1,'SampleTime',-1,'Signal',struct('SgnName',['RX signal'],'SgnStartBit',0,'SgnLength',8,'SgnType','standard','ModeValue',-1,'DataType',['unsigned int'],'ByteLayout',['little endian'],'SLDataType','SS_DOUBLE','Factor',1,'Offset',0),'StatusSelected','yes','TimeSelected','yes','DeltaTimeSelected','yes','BytePortSelected','no','MessageLengthSelected','no','EnablePortSelected','no','UserCoding',struct('Selected','no','InterfaceFile','UserDecodingFile','FcnName','UserDecodeFcn','InportSelected','no','InportWidth',1,'OutportSelected','no','OutportWidth',1),'TriggerPort',struct('Selected','no','TriggerType','rising'),'UseRXService','no','BoardType','DS4302','BoardNo',1,'ControllerNo',1,'SFcnPortType','Scalar'),'TLCFileName','rtican_rx_message')
      settings: AttributesFormatString=Group Id: RTICAN1\n
  MDPS3_CAN : Outport
  wires:
  Bus Creator/1 -> MDPS3_CAN/1  "MDPS3_CAN"
  L_MDPS3/1 -> Bus Creator/1  "CF_Mdps_MsgCount3"
  L_MDPS3/2 -> Bus Creator/2  "CR_Mdps_StrColTq"
  L_MDPS3/3 -> Bus Creator/3  "CF_Mdps_ToiFlt"
  L_MDPS3/4 -> Bus Creator/4  "CF_Mdps_ToiActive"
  L_MDPS3/5 -> Bus Creator/5  "CF_Mdps_FailStat"
  L_MDPS3/6 -> Bus Creator/6  "CF_Mdps_ToiUnavail"
  L_MDPS3/7 -> Bus Creator/7  "CF_Mdps_Chksum3"

== system Control_test/InputProcessing/VehicleCanProcessing/MDPS3Processing ==
  In1 : Inport
  Bus Creator10 : BusCreator  Inputs=5
  Bus Selector10 : BusSelector  OutputSignals=CR_Mdps_StrColTq,CF_Mdps_ToiUnavail,CF_Mdps_ToiActive,CF_Mdps_ToiFlt,CF_Mdps_FailStat
  MDPS3 Processing : Subsystem
  Out1 : Outport
  wires:
  In1/1 -> Bus Selector10/1
  Bus Creator10/1 -> Out1/1  "MDPS3Data"
  Bus Selector10/1 -> MDPS3 Processing/1(CR_Mdps_StrColTq_CAN)  "<CR_Mdps_StrColTq>"
  Bus Selector10/2 -> MDPS3 Processing/2(CR_Mdps_ToiUnavail_CAN)  "<CF_Mdps_ToiUnavail>"
  Bus Selector10/3 -> MDPS3 Processing/3(CR_Mdps_ToiActive_CAN)  "<CF_Mdps_ToiActive>"
  Bus Selector10/4 -> MDPS3 Processing/4(CR_Mdps_ToiFit_CAN)  "<CF_Mdps_ToiFlt>"
  Bus Selector10/5 -> MDPS3 Processing/5(CR_Mdps_FailStat_CAN)  "<CF_Mdps_FailStat>"
  MDPS3 Processing/1(ipMdpsStrColTq) -> Bus Creator10/1
  MDPS3 Processing/2(ipMdpsToiUnavail) -> Bus Creator10/2
  MDPS3 Processing/3(ipMdpsToiActive) -> Bus Creator10/3
  MDPS3 Processing/4(ipMdpsToiFit) -> Bus Creator10/4
  MDPS3 Processing/5(ipMdpsFailStat) -> Bus Creator10/5

== system Control_test/InputProcessing/VehicleCanProcessing/SAS1 ==
  Bus Creator : BusCreator  Inputs=5
  L_SAS1 : rtican/RTICAN Receive (RX)   Reserved1=[]  Reserved2=[]  Reserved3=[]  Reserved4=[]  SfcnMessage=[]  Msg_Struct=[]  BoardTypeNo=[]  BoardNo=[]  ChannelNo=[]  Parameters=[]  DialogFcn=[]  UnitName=[]  Revision=[]  UnitValues=[]  DSProperties=struct('RTI',struct('Version',uint32(5),'BlockType',struct('isSLSource',uint8(1),'isSLSink',uint8(1),'isHWSource',uint8(0),'isHWSink',uint8(0),'isSetup',uint8(0),'isInline',uint8(1),'isNonInline',uint8(0),'isInterrupt',uint8(0),'isChannelwise',uint8(0)),'IOBoardType','RTICAN','UnitType','MESSAGE','Identifier','RX','DialogType','MSVC','BlockSet','RTICAN','SlaveProcessor','CAN'))  RTIBlockInterface=struct('OutputPortsWidth',int32([1 1 1 1 1]),'OutputPortsActive',[1 1 1 1 1],'OutputPortsName',{{'SAS_Speed','SAS_Angle','CheckSum','MsgCount','SAS_Stat'}},'OutputPortsDataType',{{'SS_DOUBLE','SS_DOUBLE','SS_DOUBLE','SS_DOUBLE','SS_DOUBLE'}},'OutputPortsLabel',{{'SAS_Speed','SAS_Angle','CheckSum','MsgCount','SAS_Stat'}},'OutputPortsLabelMode','ON','InputPortsWidth',int32(0),'InputPortsActive',0,'DialogFcn','rtican_message_interface_gui','BlockDisplay',{{'','center'}},'IconTransparency','on','ParameterTunableNames',{{}},'InitLevel',3,'BlockName',struct('Token',{{'L_SAS1'}}),'SampleTime',{{-1}},'TriggerPort',{{'none'}},'EnablePort',{{'none'}})  RTIBlockParameters=struct('BoardTypeNo',{{1,'OFF',[]}},'BoardNo',{{1,'ON',[1 16]}},'ChannelNo',{{1,'ON',[1 2]}},'Parameters',{{struct('DataFileSupport',struct('DataFileSelectedMaster',1,'DataFileSelectedLocal',1,'DataFileName','c:\users\mpc_car\documents\github\mpc-car\controller\dbcfiles\hmc_can_for_ucb_v1.dbc|','DataFileDate',['21-Nov-2014 13:30:51'],'SelectedFile','c:\users\mpc_car\documents\github\mpc-car\dbcfiles\hmc_can_for_ucb_v2.dbc','InterfaceFcn','rtican_dbc_file_parser'),'Options',struct('StatusSelected',0,'TimeSelected',0,'DeltaTimeSelected',0,'BytePortSelected',0,'MessageLengthSelected',0,'TriggerPort',struct('Selected',0,'TriggerType',0),'UserCoding',struct('Selected',0,'InterfaceFile','UserDecodingFile','FcnName','UserDecodeFcn','InportSelected',0,'InportWidth',1,'OutportSelected',0,'OutportWidth',1),'EnablePortSelected',0,'SignalOnPortnameSelected',1,'UseRXService',0),'Message',struct('MsgOnBlocknameSelected',1,'MsgName','L_SAS1','MsgIdFormat',0,'MsgId',519,'MsgLength',5,'NumSignals',5,'SampleTime',-1,'Signal',struct('SgnName',{'SAS_Speed','SAS_Angle','CheckSum','MsgCount','SAS_Stat'},'SgnStartBit',{0,8,24,28,32},'SgnLength',{8,16,4,4,8},'ByteLayout',{0,0,0,0,0},'Factor',{4,0.1,1,1,1},'Offset',{0,0,0,0,0},'SgnComment',{['When MDPS ECU sends this message, this message value is valid 1.5 sec later from IG-ON.'],['When MDPS ECU sends this message, this message value is valid 1.5 sec later from IG-ON.'],['When MDPS ECU sends this message, this message value is valid 1.5 sec later from IG-ON.'],['When MDPS ECU sends this message, this message value is valid 1.5 sec later from IG-ON.'],['When MDPS ECU sends this message, this message value is valid 1.5 sec later from IG-ON.']},'SgnUnit',{'','Degree','','',''},'Min',{0,-3276.8,0,0,0},'Max',{1016,3276.7,15,15,255},'SgnType',{0,0,0,0,0},'SLDataType',{'SS_DOUBLE','SS_DOUBLE','SS_DOUBLE','SS_DOUBLE','SS_DOUBLE'},'DataType',{0,1,0,0,0},'ModeValue',{-1,-1,-1,-1,-1}),'MsgIdNumFormat',0,'MsgComment',{{''}}),'Version',1.2,'general',struct('isFromLib',0)),'OFF',[]}},'GroupId',{{struct('Group',{{'RTICAN'}},'No',1,'Behavior',{{'NAMECHANGE'}},'BlockType',{{'SINK'}},'NameChangeFlag',0),'OFF',[]}},'SFcnRTICANMessage',{{struct('MsgType','RX','SFcnPortType','Scalar','MsgName','L_SAS1','MsgIdFormat','STD','MsgId',519,'MsgLength',5,'NumSignals',5,'SampleTime',-1,'Signal',struct('SgnName',{'SAS_Speed','SAS_Angle','CheckSum','MsgCount','SAS_Stat'},'SgnStartBit',{0,8,24,28,32},'SgnLength',{8,16,4,4,8},'ByteLayout',{['little endian'],['little endian'],['little endian'],['little endian'],['little endian']},'Factor',{4,0.1,1,1,1},'Offset',{0,0,0,0,0},'SgnType',{'standard','standard','standard','standard','standard'},'SLDataType',{'SS_DOUBLE','SS_DOUBLE','SS_DOUBLE','SS_DOUBLE','SS_DOUBLE'},'DataType',{['unsigned int'],['signed int'],['unsigned int'],['unsigned int'],['unsigned int']},'ModeValue',{-1,-1,-1,-1,-1}),'StatusSelected','no','TimeSelected','no','DeltaTimeSelected','no','BytePortSelected','no','MessageLengthSelected','no','TriggerPort',struct('Selected','no','TriggerType',0),'UserCoding',struct('Selected','no','InterfaceFile','UserDecodingFile','FcnName','UserDecodeFcn','InportSelected','no','InportWidth',1,'OutportSelected','no','OutportWidth',1),'EnablePortSelected','no','UseRXService','no','BoardType','DS1','BoardNo',1,'ControllerNo',1),'OFF',[]}},'TLCFileName',{{'rtican_rx_message','OFF',[]}})  RTISFcnParameters=struct('SFcnRTICANMessage','struct','TLCFileName','char')  RTIBlockParaDefault=struct('BoardTypeNo',4302,'BoardNo',1,'ChannelNo',1,'Parameters',struct('DataFileSupport',struct('DataFileSelectedMaster',0,'DataFileSelectedLocal',0,'DataFileName','','DataFileDate','','SelectedFile',['<no file selected>']),'Options',struct('StatusSelected',1,'TimeSelected',1,'DeltaTimeSelected',1,'BytePortSelected',0,'MessageLengthSelected',0,'TriggerPort',struct('Selected',0,'TriggerType','rising'),'UserCoding',struct('Selected',0,'InterfaceFile','UserDecodingFile','FcnName','UserDecodeFcn','InportSelected',0,'InportWidth',1,'OutportSelected',0,'OutportWidth',1),'EnablePortSelected',0,'SignalOnPortnameSelected',1,'UseRXService',0),'Message',struct('MsgOnBlocknameSelected',0,'MsgName',['RX Message'],'MsgIdFormat',0,'MsgId',100,'MsgLength',8,'NumSignals',1,'SampleTime',-1,'Signal',struct('SgnName',['RX signal'],'SgnStartBit',0,'SgnLength',8,'SgnType',0,'ModeValue',-1,'DataType',0,'SLDataType','SS_DOUBLE','ByteLayout',0,'Factor',1,'Offset',0,'Min',0,'Max',255,'SgnComment',{{}},'SgnUnit',''),'MsgIdNumFormat',0,'MsgComment',{{''}}),'Version',1.2,'general',struct('isFromLib',1)),'GroupId',struct('Group',{{'RTICAN'}},'No',1,'Behavior',{{'NAMECHANGE'}},'BlockType',{{'SINK'}},'NameChangeFlag',0),'SFcnRTICANMessage',struct('MsgType','RX','MsgName',['RX Message'],'MsgIdFormat','STD','MsgId',100,'MsgLength',8,'NumSignals',1,'SampleTime',-1,'Signal',struct('SgnName',['RX signal'],'SgnStartBit',0,'SgnLength',8,'SgnType','standard','ModeValue',-1,'DataType',['unsigned int'],'ByteLayout',['little endian'],'SLDataType','SS_DOUBLE','Factor',1,'Offset',0),'StatusSelected','yes','TimeSelected','yes','DeltaTimeSelected','yes','BytePortSelected','no','MessageLengthSelected','no','EnablePortSelected','no','UserCoding',struct('Selected','no','InterfaceFile','UserDecodingFile','FcnName','UserDecodeFcn','InportSelected','no','InportWidth',1,'OutportSelected','no','OutportWidth',1),'TriggerPort',struct('Selected','no','TriggerType','rising'),'UseRXService','no','BoardType','DS4302','BoardNo',1,'ControllerNo',1,'SFcnPortType','Scalar'),'TLCFileName','rtican_rx_message')
      settings: AttributesFormatString=Group Id: RTICAN1\n
  SAS1_CAN : Outport
  wires:
  Bus Creator/1 -> SAS1_CAN/1  "SAS1_CAN"
  L_SAS1/1 -> Bus Creator/1  "SAS_Speed"
  L_SAS1/2 -> Bus Creator/2  "SAS_Angle"
  L_SAS1/3 -> Bus Creator/3  "CheckSum"
  L_SAS1/4 -> Bus Creator/4  "MsgCount"
  L_SAS1/5 -> Bus Creator/5  "SAS_Stat"

== system Control_test/InputProcessing/VehicleCanProcessing/SAS1Processing ==
  In1 : Inport
  Bus Creator4 : BusCreator  Inputs=6
  Bus Selector4 : BusSelector  OutputSignals=SAS_Angle,SAS_Speed,MsgCount,CheckSum
  SAS1 Processing : Subsystem
  Out1 : Outport
  wires:
  Bus Selector4/1 -> SAS1 Processing/1(SAS_Angle_CAN)  "<SAS_Angle>"
  Bus Selector4/2 -> SAS1 Processing/2(SAS_Speed_CAN)  "<SAS_Speed>"
  Bus Selector4/3 -> SAS1 Processing/3(MsgCount_CAN)  "<MsgCount>"
  Bus Selector4/4 -> SAS1 Processing/4(CheckSum_CAN)  "<CheckSum>"
  SAS1 Processing/1(ipStrAng [deg]) -> Bus Creator4/1
  SAS1 Processing/2(ipStrAngEr) -> Bus Creator4/2
  SAS1 Processing/3(ipStrSpd [deg/s]) -> Bus Creator4/3
  SAS1 Processing/4(ipStrSpdEr) -> Bus Creator4/4
  SAS1 Processing/5(ipSasCnt) -> Bus Creator4/5
  SAS1 Processing/6(ipSasCksum) -> Bus Creator4/6
  Bus Creator4/1 -> Out1/1  "SAS1Data"
  In1/1 -> Bus Selector4/1
